simulink model "phi2_m1_vr01_k2_2"  (R2021a)
settings: Solver=FixedStepAuto  StartTime=0.0  StopTime=24.0  FixedStep=1.0  RelTol=1e-3
libraries: deeplib x1
settings Model: Creator=ldy  LastModifiedBy=ldy
settings DataIOCC: SaveFormat=Array  SignalLogging=off  DSMLogging=off
settings DebuggingCC: UnconnectedInputMsg=none  UnconnectedOutputMsg=none  UnconnectedLineMsg=none
settings ModelReferenceCC: EnableRefExpFcnMdlSchedulingChecks=off
settings RTWCC: Description=Generic Real-Time Target  GPUComputeCapability=5.0  DLArmComputeVersion=20.02.1

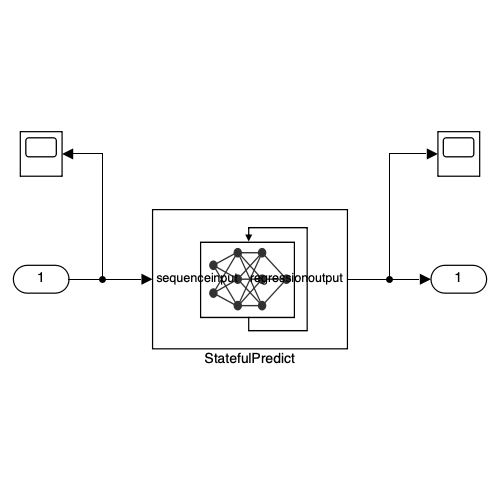
[thumbnail: Simulink's stored preview of the top-level diagram]
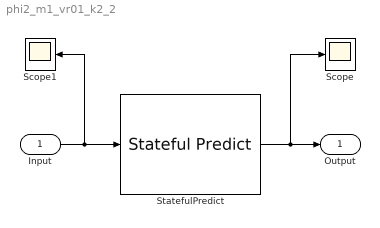
== system phi2_m1_vr01_k2_2 ==
  Input : Inport
  Scope : Scope
  Scope1 : Scope
  StatefulPredict : deeplib/Stateful Predict  Network=Network from MAT-file  NetworkFunction=untitled  NetworkFilePath=SB2-Synthetic_Benchmark_2/phi2_m1_vr01_k2_2.mat  InputDataFormats={'',''}  SampleTime=1  ForceInterpretedSim=off  EnableDLNetwork=on  LastKnownNetworkFilePath=''  LastKnownNetworkTimeStamp=''
  Output : Outport
  wires:
  Input/1 -> Scope1/1, StatefulPredict/1
  StatefulPredict/1 -> Scope/1, Output/1
